simulink model "P4"  (Simulink 9.3)
settings: Solver=ode45  StartTime=0.0  StopTime=tfinal  RelTol=1e-6  EnableMultiTasking=on
values from neighbouring files (symbols this model uses):
  a = g/L    (= 32.6666666667)    [P4_1.m]    (also in P4_2_1.m; P4_2_2.m; P4_2_3.m; P4_3.m)
  b = k/m    (= 0.1)    [P4_1.m]    (also in P4_2_1.m; P4_2_2.m; P4_2_3.m; P4_3.m)
  c = 1/(m*L^2)    (= 111.111111111)    [P4_1.m]    (also in P4_2_1.m; P4_2_2.m; P4_2_3.m; P4_3.m)
  h = 0.1    [P4_1.m]    (also in P4_2_1.m; P4_2_2.m; P4_2_3.m; P4_3.m)
  md = MPCInit(Ad,Bd,Cyd,Czd,Dzd,Ccd,Dcd,Hp,Hw,zblk,Hu,ublk,  	    du_max,du_min,u_max,u_min,z_max,  	    z_min,Q,R,W,V,h,cmode,solver)    [P4_1.m]    (also in P4_2_1.m = MPCInit(Ad,Bd,Cyd,Czd,Dzd,Ccd,Dcd,Hp,Hw,zblk,Hu,ublk,  	    ; P4_2_2.m = MPCInit(Ad,Bd,Cyd,Czd,Dzd,Ccd,Dcd,Hp,Hw,zblk,Hu,ublk,  	    ; P4_2_3.m = MPCInit(Ad,Bd,Cyd,Czd,Dzd,Ccd,Dcd,Hp,Hw,zblk,Hu,ublk,  	    ; P4_3.m = MPCInit(Ad,Bd,Cyd,Czd,Dzd,Ccd,Dcd,Hp,Hw,zblk,Hu,ublk,  	    )
settings Model: Creator=jakesson  LastModifiedBy=tomas  ExtModeAutoUpdateStatusClock=off
settings DataIOCC: LimitDataPoints=on  SignalLoggingName=sigsOut
settings OptimizationCC: BooleanDataType=off  InitFltsAndDblsToZero=on
settings DebuggingCC: SaveWithParameterizedLinksMsg=none  SignalResolutionControl=TryResolveAllWithWarning  MultiTaskDSMMsg=warning  MultiTaskCondExecSysMsg=none
settings HardwareCC: TargetUnknown=on
settings GRTTargetCC: TargetFcnLib=ansi_tfl_tmw.mat  GeneratePreprocessorConditionals=Disable all

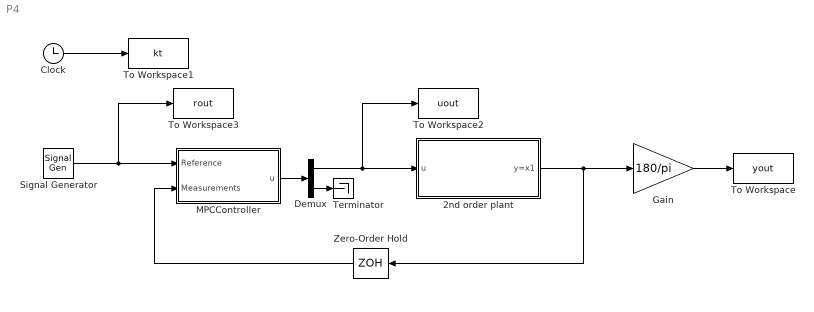
== system P4 ==
  2nd order plant : Subsystem
  Clock : Clock
  Demux : Demux  Outputs=[md.m md.ne]
  Gain : Gain  Gain=180/pi
  MPCController : Subsystem  mask{md=md}
      mask prompts: md "MPCData"
  Signal Generator : SignalGenerator  WaveForm=square  Amplitude=0  Units=rad/sec
  Terminator : Terminator
  To Workspace : ToWorkspace  VariableName=yout  SampleTime=-1
  To Workspace1 : ToWorkspace  VariableName=kt  SampleTime=-1
  To Workspace2 : ToWorkspace  VariableName=uout  SampleTime=-1
  To Workspace3 : ToWorkspace  VariableName=rout  SampleTime=-1
  Zero-Order Hold : ZeroOrderHold  SampleTime=h
  wires:
  Demux/2 -> Terminator/1
  MPCController/1(u) -> Demux/1
  Clock/1 -> To Workspace1/1
  Demux/1 -> 2nd order plant/1(u), To Workspace2/1
  Signal Generator/1 -> To Workspace3/1, MPCController/1(Reference)
  2nd order plant/1(y=x1) -> Zero-Order Hold/1, Gain/1
  Zero-Order Hold/1 -> MPCController/2(Measurements)
  Gain/1 -> To Workspace/1

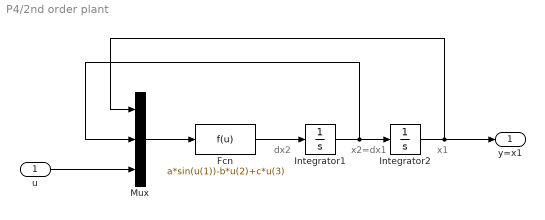
== system P4/2nd order plant ==
  note: x2=dx1
  note: dx2
  note: x1
  u : Inport
  Fcn : Fcn  Expr=a*sin(u(1))-b*u(2)+c*u(3)
  "Integrator1 " : Integrator
  "Integrator2 " : Integrator  InitialCondition=20*pi/180
  Mux : Mux  Inputs=3
  y=x1 : Outport
  wires:
  u/1 -> Mux/3
  Mux/1 -> Fcn/1
  "Integrator1 "/1 -> Mux/2, "Integrator2 "/1
  Fcn/1 -> "Integrator1 "/1
  "Integrator2 "/1 -> y=x1/1, Mux/1

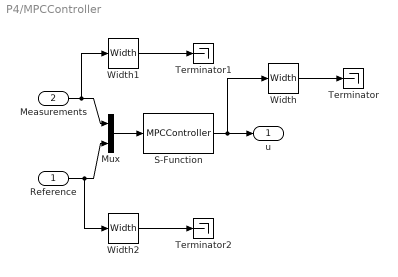
== system P4/MPCController ==
  Reference : Inport
  Measurements : Inport  Port=2
  Mux : Mux  Inputs=2
  S-Function : S-Function  FunctionName=MPCController  Parameters=md  SFunctionDeploymentMode=off  EnableBusSupport=off
  Terminator : Terminator
  Terminator1 : Terminator
  Terminator2 : Terminator
  Width : Width
  Width1 : Width
  Width2 : Width
  u : Outport
  wires:
  Mux/1 -> S-Function/1
  Measurements/1 -> Width1/1, Mux/1
  Reference/1 -> Width2/1, Mux/2
  S-Function/1 -> Width/1, u/1
  Width/1 -> Terminator/1
  Width1/1 -> Terminator1/1
  Width2/1 -> Terminator2/1
